simulink model "controlMCUSlugsMKII"  (Simulink 6.6)
settings: Solver=FixedStepDiscrete  StartTime=0.0  StopTime=10.0  FixedStep=0.01  RelTol=1e-3
InitFcn:
  | mcuInit
values from neighbouring files (symbols this model uses):
  apSampleTime = 0.01    [mcuInit.m]
  derivativesConstant = 5    [mcuInit.m]
  T = 0.01    [mcuInit.m]
undefined symbols (not defined in the file or in its folder): bankCommandLimit, baseHeight, bda, bde, bdr, bdt, bICda, bICde, bICdr, bICdt, controlMCUInit, daLimit, deLimit, drLimit, dtLimit, getAccBias, getAccels, getAttitude, getMidLevelCommands, getPassValues, getPidIdx, getVned, getWP, getXYZ, gsRead, ISA_g, lowRateTelemetryMavlink, mda, mde, mdr, mdt, mICda, mICde, mICdr, mICdt, pitchCommandLimit, protDecodeMavlink, readIpc, send2GS, setCurrentCommands, setDiagnosticFloat, setDiagnosticShort, setLogFloat1, setLogFloat2, setNavLat, setNavLong, setNavNav, u1, u2, updateEuler, updateLoad, updatePQR, updatePWM, updatePWM2, y1
libraries: dsPICdrivers x85, simulink x79, SLUGS_Library x23, aerolibconvert2 x5, aerolibutil x3
(part 1 of 5)
settings Model: Creator=ASL_Lab  LastModifiedBy=Administrator  ProdHWDeviceType=16-bit Generic
settings OptimizationCC: InlineParams=on  OptimizeModelRefInitCode=on  LifeSpan=1
settings HardwareCC: ProdBitPerInt=16  ProdEndianess=LittleEndian  ProdWordSize=16  ProdHWDeviceType=16-bit Generic  TargetHWDeviceType=32-bit Generic
settings RTWCC: SystemTargetFile=dspic.tlc  TemplateMakefile=dspic_pic30_gcc.tmf  PostCodeGenCommand=dsPIC_Compile()  Description=Embedded Target for Microchip dsPIC (real-time)  GenerateReport=on  ProcessScript=dspic_make_rtw_hook  CustomInclude=..\mavlink\include\slugs\  IncludeHyperlinkInReport=on  LaunchReport=on
settings RTWCC: CustomSource=|
  | clib\circBuffer.c
  | clib\sbrk.c
  | clib\interProcCommSlave.c
  | clib\eepLoader.c
  | clib\apUtils.c
  | clib\DEE.c
  | clib\DEES.s
  | clib\navSupport.c
  | clib\mavlinkControlMcu.c
  | clib\updateControlMcuState.c
  | clib\mavlinkCommsControlMcu.c
settings CodeAppCC: IgnoreCustomStorageClasses=off
settings STFCustomTargetCC: TargetFcnLib=ansi_tfl_tmw.mat  GenFloatMathFcnCalls=ANSI_C  ModelReferenceCompliant=off  IncludeMdlTerminateFcn=off  CombineOutputUpdateFcns=on  SuppressErrorStatus=on  ERTCustomFileBanners=on  SupportContinuousTime=off  SupportNonInlinedSFcns=off  SystemTargetFile=dspic.tlc
settings ERTTargetCC: TargetFcnLib=ansi_tfl_tmw.mat  GenFloatMathFcnCalls=ANSI_C  ModelReferenceCompliant=off  IncludeMdlTerminateFcn=off  SuppressErrorStatus=on  ModelStepFunctionPrototypeControlCompliant=off  ExtModeMexFile=noextcomm  InlinedParameterPlacement=NonHierarchical  ERTSrcFileBannerTemplate=dsPIC_code_template.cgt  ERTHdrFileBannerTemplate=dsPIC_code_template.cgt  ERTDataSrcFileTemplate=dsPIC_code_template.cgt  ERTDataHdrFileTemplate=dsPIC_code_template.cgt  ERTCustomFileTemplate=dsPIC_main.tlc
settings CustomProperty: DataType=string  Value=C:\PROGRA~1\MATLAB\R2007a\rtw\bin\win32\gmake

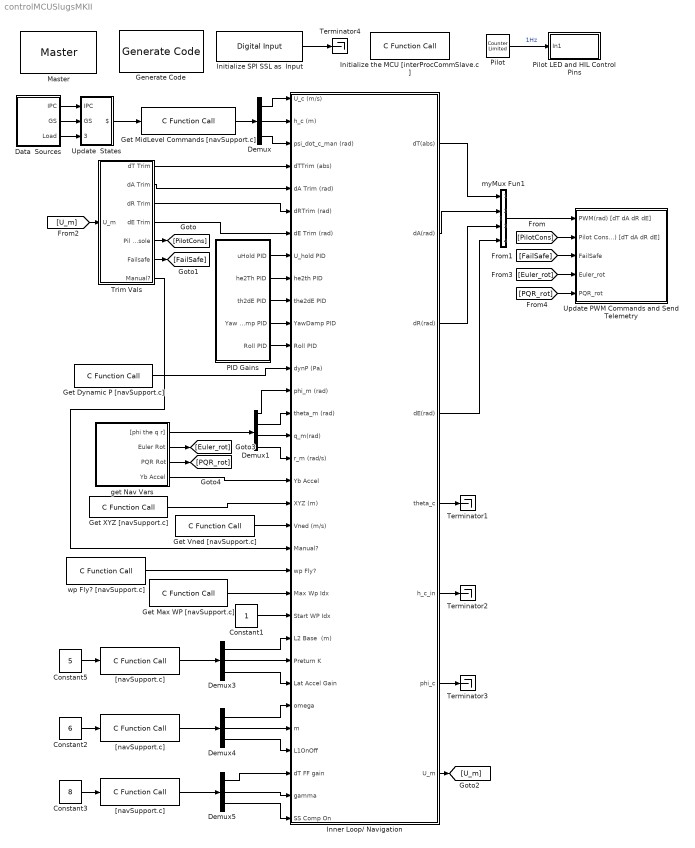
== system controlMCUSlugsMKII ==
  Constant1 : Constant  OutDataTypeMode=uint8
  Constant2 : Constant  Value=6  OutDataTypeMode=uint8
  Constant3 : Constant  Value=8  OutDataTypeMode=uint8
  Constant5 : Constant  Value=5  OutDataTypeMode=uint8
  Data  Sources : Subsystem
  Demux{,3..5} (4 alike) : Demux  Outputs=3
  Demux1 : Demux
  Generate Code : dsPICdrivers/Simulink Configuration/Generate Code
  Get Dynamic P [navSupport.c] : dsPICdrivers/OTHERS/C Function Call  Tag=dsPIC_dsPIC_CFunctionCall  fctName='getDynamic'  INPUT_SIZE=1  INPUT1=--  INPUT2=--  INPUT3=--  OUTPUT_SIZE=1  OUTPUT1=real32  SampleTime=.01  InputType=[ ]  OutputType=[ 7 ]  FctDeclaration=extern real32_T getDynamic();  FctCall=%y1 = getDynamic();  OrderingInOutPopup=None
  Get Max WP [navSupport.c] : dsPICdrivers/OTHERS/C Function Call  Tag=dsPIC_dsPIC_CFunctionCall  fctName='getMaxWp'  INPUT_SIZE=1  INPUT1=--  INPUT2=--  INPUT3=--  OUTPUT_SIZE=1  OUTPUT1=uint8  SampleTime=.01  InputType=[ ]  OutputType=[ 2 ]  FctDeclaration=extern uint8_T getMaxWp();  FctCall=%y1 = getMaxWp();  OrderingInOutPopup=None
  Get MidLevel Commands [navSupport.c] : dsPICdrivers/OTHERS/C Function Call  Tag=dsPIC_dsPIC_CFunctionCall  fctName='getMidLevelCommands'  INPUT_SIZE=1  INPUT1=--  INPUT2=--  INPUT3=--  OUTPUT_SIZE=3  OUTPUT1=real32  SampleTime=.01  InputType=[ ]  OutputType=[ 7 ]  FctDeclaration=extern void getMidLevelCommands(real32_T* y1);  FctCall=getMidLevelCommands(*%y1);  OrderingInOutPopup=Input
  Get Vned [navSupport.c] : dsPICdrivers/OTHERS/C Function Call  Tag=dsPIC_dsPIC_CFunctionCall  fctName='getVned'  INPUT_SIZE=1  INPUT1=--  INPUT2=--  INPUT3=--  OUTPUT_SIZE=3  OUTPUT1=real32  SampleTime=.01  InputType=[ ]  OutputType=[ 7 ]  FctDeclaration=extern void getVned(real32_T* y1);  FctCall=getVned(*%y1);  OrderingInOutPopup=None
  Get XYZ [navSupport.c] : dsPICdrivers/OTHERS/C Function Call  Tag=dsPIC_dsPIC_CFunctionCall  fctName='getXYZ'  INPUT_SIZE=1  INPUT1=--  INPUT2=--  INPUT3=--  OUTPUT_SIZE=3  OUTPUT1=real32  SampleTime=.01  InputType=[ ]  OutputType=[ 7 ]  FctDeclaration=extern void getXYZ(real32_T* y1);  FctCall=getXYZ(*%y1);  OrderingInOutPopup=None
  Initialize SPI SSL as  Input : dsPICdrivers/Digital I//O/Digital Input  Tag=dsPIC_Digital_Input  PORT=B  Pin=[2]  SampleTime=inf  OrderingInOutPopup=None
  Initialize the MCU [interProcCommSlave.c] : dsPICdrivers/OTHERS/C Function Call  Tag=dsPIC_dsPIC_CFunctionCall  fctName='controlMCUInit'  INPUT_SIZE=1  INPUT1=--  INPUT2=--  INPUT3=--  OUTPUT_SIZE=1  OUTPUT1=--  SampleTime=inf  InputType=[ ]  OutputType=[ ]  FctDeclaration=extern void controlMCUInit();  FctCall=controlMCUInit();  OrderingInOutPopup=None
  Inner Loop/ Navigation : Subsystem
  Master : dsPICdrivers/Master  Tag=dsPIC_MASTER  Priority=1  TimeStepType=Timer1  picType=33fJ256MC710  fcy=40000000  Quartz_33f=12e6  PLLActive_33f=on  fcyDesired_33f=40e6  tmr1="[8  49999  0]"  tmr1Info="Time Step : 0.01  ;   Error : 0%  PR1=49999"  tmr2345="[8  0  0  0  0  0  0  0]"  tmr2345cfg=[-1 -1 -1 -1 -1 -1 -1 -1]  IOautoConf=on  typePort="[ 0   0   0   0   0   0   0   0   0   0   0   0   0   0   0   0   0   0   9   0   0   0  10   0   0   0   0   0   0   0   0   0   0   0   0   0   0   0   0   0   0   0   0   0   0   0   0   0   0   0   0   0   0   0   0   0   0   6   6   6   6   0   0   6  11   0  11   0  11   0  11   0   0  10   0   0   0   0   0   0   0   0   0   0   0   0   0   0   0   0   0   0   0   0   0   0   0   0   0   0   0   0   0   0   0   0   0   0   0   0   0   0 ]"  TRIS="[ 65535  65471  65535  65535  65023  65535  65535 ]"  ADPCFG=2097220  MasterBusyPort=None  MasterOverloadPort=None  FOSC=External Clock  ClockSwitchMonitor=Both disabled  TempProtection_33f=TEMP_ON  FPBOR=<empty>  PWRT=64ms  MCLR=<empty>  PowerSave=off  OverrideFcy=off  NewFcy=1e6  PR2345="[65535  65535  65535  65535  65535  65535  65535  65535]"
  PID Gains : Subsystem
  Pilot : simulink/Sources/Counter Limited  SystemSampleTime=-1  uplimit=1  tsamp=1.0
  Pilot LED and HIL Control Pins : Subsystem
  Terminator{1..4} (4 alike) : Terminator
  Trim Vals : Subsystem
  Update  States : Subsystem
  Update PWM Commands and Send Telemetry : Subsystem
  "[navSupport.c]" : dsPICdrivers/OTHERS/C Function Call  Tag=dsPIC_dsPIC_CFunctionCall  fctName='getPidIdx'  INPUT_SIZE=1  INPUT1=uint8  INPUT2=--  INPUT3=--  OUTPUT_SIZE=3  OUTPUT1=real32  SampleTime=.01  InputType=[ 2 ]  OutputType=[ 7 ]  FctDeclaration=extern void getPidIdx(uint8_T u1,real32_T* y1);  FctCall=getPidIdx(%u1, *%y1);  OrderingInOutPopup=None
  "[navSupport.c] " : dsPICdrivers/OTHERS/C Function Call  Tag=dsPIC_dsPIC_CFunctionCall  fctName='getPidIdx'  INPUT_SIZE=1  INPUT1=uint8  INPUT2=--  INPUT3=--  OUTPUT_SIZE=3  OUTPUT1=real32  SampleTime=.01  InputType=[ 2 ]  OutputType=[ 7 ]  FctDeclaration=extern void getPidIdx(uint8_T u1,real32_T* y1);  FctCall=getPidIdx(%u1, *%y1);  OrderingInOutPopup=None
  "[navSupport.c]   " : dsPICdrivers/OTHERS/C Function Call  Tag=dsPIC_dsPIC_CFunctionCall  fctName='getPidIdx'  INPUT_SIZE=1  INPUT1=uint8  INPUT2=--  INPUT3=--  OUTPUT_SIZE=3  OUTPUT1=real32  SampleTime=.01  InputType=[ 2 ]  OutputType=[ 7 ]  FctDeclaration=extern void getPidIdx(uint8_T u1,real32_T* y1);  FctCall=getPidIdx(%u1, *%y1);  OrderingInOutPopup=None
  get Nav Vars : Subsystem
  myMux Fun1 : Stateflow chart
  wp Fly? [navSupport.c] : dsPICdrivers/OTHERS/C Function Call  Tag=dsPIC_dsPIC_CFunctionCall  fctName='isWpFly'  INPUT_SIZE=1  INPUT1=--  INPUT2=--  INPUT3=--  OUTPUT_SIZE=1  OUTPUT1=uint8  SampleTime=.01  InputType=[ ]  OutputType=[ 2 ]  FctDeclaration=extern uint8_T isWpFly();  FctCall=%y1 = isWpFly();  OrderingInOutPopup=None
  wires:
  Pilot/1 -> Pilot LED and HIL Control Pins/1(In1)  "1Hz"
  Initialize SPI SSL as  Input/1 -> Terminator4/1
  Data  Sources/1(IPC) -> Update  States/1(IPC)
  Data  Sources/2(GS) -> Update  States/2(GS)
  Data  Sources/3(Load) -> Update  States/3(Load)
  Demux/1 -> Inner Loop/ Navigation/1(U_c (m/s))
  Demux/2 -> Inner Loop/ Navigation/2(h_c (m))
  Demux/3 -> Inner Loop/ Navigation/3(psi_dot_c_man (rad))
  Get MidLevel Commands [navSupport.c]/1 -> Demux/1
  Trim Vals/4(dE Trim) -> Inner Loop/ Navigation/7(dE Trim (rad))
  Trim Vals/1(dT Trim) -> Inner Loop/ Navigation/4(dTTrim (abs))
  Trim Vals/2(dA Trim) -> Inner Loop/ Navigation/5(dA Trim (rad))
  Trim Vals/3(dR Trim) -> Inner Loop/ Navigation/6(dRTrim (rad))
  PID Gains/1(uHold PID) -> Inner Loop/ Navigation/8(U_hold PID)
  PID Gains/2(he2Th PID) -> Inner Loop/ Navigation/9(he2th PID)
  PID Gains/3(th2dE PID) -> Inner Loop/ Navigation/10(the2dE PID)
  PID Gains/4(Yaw Damp PID) -> Inner Loop/ Navigation/11(YawDamp PID)
  PID Gains/5(Roll PID) -> Inner Loop/ Navigation/12("Roll PID ")
  Constant1/1 -> Inner Loop/ Navigation/24(Start WP Idx)
  Get Dynamic P [navSupport.c]/1 -> Inner Loop/ Navigation/13(dynP (Pa))
  get Nav Vars/1("[phi the q r]") -> Demux1/1
  Demux1/1 -> Inner Loop/ Navigation/14(phi_m (rad))
  Demux1/2 -> Inner Loop/ Navigation/15(theta_m (rad))
  Get Max WP [navSupport.c]/1 -> Inner Loop/ Navigation/23(Max Wp Idx)
  Update  States/1($) -> Get MidLevel Commands [navSupport.c]/1
  Trim Vals/7(Manual?) -> Inner Loop/ Navigation/21(Manual?)
  wp Fly? [navSupport.c]/1 -> Inner Loop/ Navigation/22(wp Fly?)
  Inner Loop/ Navigation/5(theta_c) -> Terminator1/1
  Inner Loop/ Navigation/6(h_c_in) -> Terminator2/1
  Inner Loop/ Navigation/7(phi_c) -> Terminator3/1
  Constant5/1 -> "[navSupport.c]"/1
  "[navSupport.c]"/1 -> Demux3/1
  Demux3/1 -> Inner Loop/ Navigation/25(L2 Base  (m))
  Demux3/2 -> Inner Loop/ Navigation/26(Preturn K)
  Demux1/4 -> Inner Loop/ Navigation/17(r_m (rad/s))
  Demux1/3 -> Inner Loop/ Navigation/16(q_m(rad))
  Demux3/3 -> Inner Loop/ Navigation/27(Lat Accel Gain)
  Constant2/1 -> "[navSupport.c] "/1
  "[navSupport.c] "/1 -> Demux4/1
  Demux4/1 -> Inner Loop/ Navigation/28(omega)
  Demux4/2 -> Inner Loop/ Navigation/29(m)
  Demux4/3 -> Inner Loop/ Navigation/30(L1OnOff)
  Trim Vals/5(Pil Console) -> [PilotCons]
  Trim Vals/6("Failsafe ") -> [FailSafe]
  Inner Loop/ Navigation/1(dT(abs)) -> myMux Fun1/1(u1)
  Inner Loop/ Navigation/2(dA(rad)) -> myMux Fun1/2(u2)
  Inner Loop/ Navigation/3(dR(rad)) -> myMux Fun1/3(u3)
  Inner Loop/ Navigation/4(dE(rad)) -> myMux Fun1/4(u4)
  [PilotCons] -> Update PWM Commands and Send Telemetry/2(Pilot Console (IC) [dT dA dR dE])
  myMux Fun1/1(y) -> Update PWM Commands and Send Telemetry/1(PWM(rad) [dT dA dR dE])
  Inner Loop/ Navigation/8(U_m) -> [U_m]
  [U_m] -> Trim Vals/1(U_m)
  [FailSafe] -> Update PWM Commands and Send Telemetry/3(FailSafe)
  get Nav Vars/2(Euler Rot) -> [Euler_rot]
  get Nav Vars/3(PQR Rot) -> [PQR_rot]
  [Euler_rot] -> Update PWM Commands and Send Telemetry/4(Euler_rot)
  [PQR_rot] -> Update PWM Commands and Send Telemetry/5(PQR_rot)
  Constant3/1 -> "[navSupport.c]   "/1
  "[navSupport.c]   "/1 -> Demux5/1
  Demux5/1 -> Inner Loop/ Navigation/31(dT FF gain)
  Demux5/2 -> Inner Loop/ Navigation/32(gamma)
  Demux5/3 -> Inner Loop/ Navigation/33(SS Comp On)
  get Nav Vars/4(Yb Accel) -> Inner Loop/ Navigation/18(Yb Accel)
  Get XYZ [navSupport.c]/1 -> Inner Loop/ Navigation/19(XYZ (m))
  Get Vned [navSupport.c]/1 -> Inner Loop/ Navigation/20(Vned (m/s))

== system controlMCUSlugsMKII/Data  Sources ==
  Compute Load : Subsystem
  Data from GS [mavlinkCommsControlMcu.c] : dsPICdrivers/OTHERS/C Function Call  Tag=dsPIC_dsPIC_CFunctionCall  fctName='gsRead'  INPUT_SIZE=1  INPUT1=--  INPUT2=--  INPUT3=--  OUTPUT_SIZE=109  OUTPUT1=uint8  SampleTime=.01  InputType=[ ]  OutputType=[ 2 ]  FctDeclaration=extern void gsRead(uint8_T* y1);  FctCall=gsRead(*%y1);  OrderingInOutPopup=None
  Data from IPC [interProcCommSlave.c] : dsPICdrivers/OTHERS/C Function Call  Tag=dsPIC_dsPIC_CFunctionCall  fctName='readIpc'  INPUT_SIZE=1  INPUT1=--  INPUT2=--  INPUT3=--  OUTPUT_SIZE=109  OUTPUT1=uint8  SampleTime=.01  InputType=[ ]  OutputType=[ 2 ]  FctDeclaration=extern void readIpc(uint8_T* y1);  FctCall=readIpc(*%y1);  OrderingInOutPopup=None
  IPC : Outport
  GS : Outport  Port=2
  Load : Outport  Port=3
  wires:
  Data from IPC [interProcCommSlave.c]/1 -> IPC/1
  Data from GS [mavlinkCommsControlMcu.c]/1 -> GS/1
  Compute Load/1(Load (%)) -> Load/1

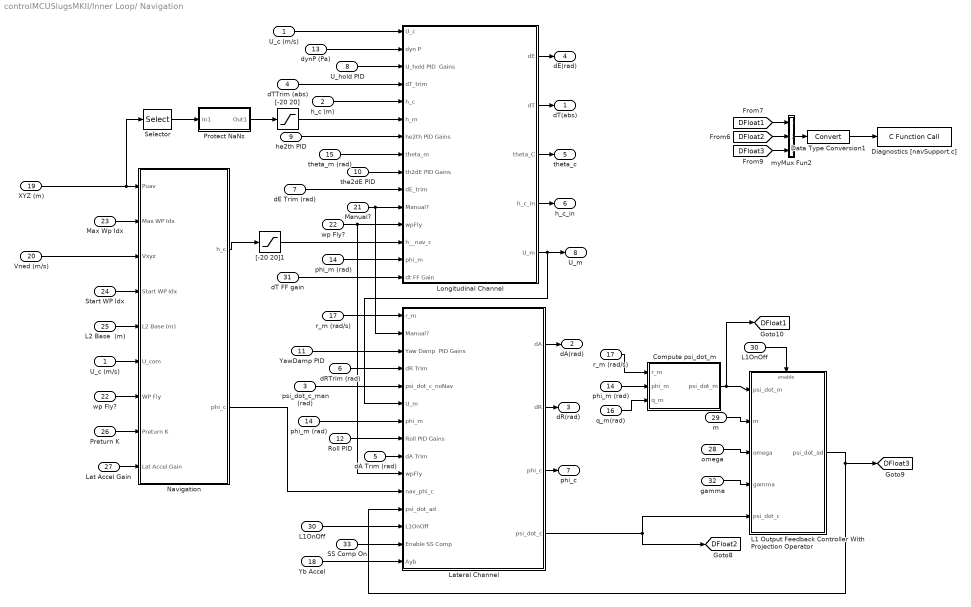
== system controlMCUSlugsMKII/Inner Loop/ Navigation ==
  U_c (m/s) : Inport
  h_c (m) : Inport  Port=2
  psi_dot_c_man (rad) : Inport  Port=3
  dTTrim (abs) : Inport  Port=4
  dA Trim (rad) : Inport  Port=5
  dRTrim (rad) : Inport  Port=6
  dE Trim (rad) : Inport  Port=7
  U_hold PID : Inport  Port=8
  he2th PID : Inport  Port=9
  the2dE PID : Inport  Port=10
  YawDamp PID : Inport  Port=11
  "Roll PID " : Inport  Port=12
  dynP (Pa) : Inport  Port=13
  phi_m (rad) : Inport  Port=14
  theta_m (rad) : Inport  Port=15
  q_m(rad) : Inport  Port=16
  r_m (rad/s) : Inport  Port=17
  Yb Accel : Inport  Port=18
  XYZ (m) : Inport  Port=19
  Vned (m/s) : Inport  Port=20
  Manual? : Inport  Port=21
  wp Fly? : Inport  Port=22
  Max Wp Idx : Inport  Port=23
  Start WP Idx : Inport  Port=24
  L2 Base  (m) : Inport  Port=25
  Preturn K : Inport  Port=26
  Lat Accel Gain : Inport  Port=27
  omega : Inport  Port=28
  m : Inport  Port=29
  L1OnOff : Inport  Port=30
  dT FF gain : Inport  Port=31
  gamma : Inport  Port=32
  SS Comp On : Inport  Port=33
  Compute psi_dot_m : Subsystem
  Data Type Conversion1 : DataTypeConversion  OutDataTypeMode=single
  Diagnostics [navSupport.c] : dsPICdrivers/OTHERS/C Function Call  Tag=dsPIC_dsPIC_CFunctionCall  fctName='setDiagnosticFloat'  INPUT_SIZE=3  INPUT1=real32  INPUT2=--  INPUT3=--  OUTPUT_SIZE=1  OUTPUT1=--  SampleTime=.01  InputType=[ 7 ]  OutputType=[ ]  FctDeclaration=extern void setDiagnosticFloat(real32_T* u1);  FctCall=setDiagnosticFloat(*%u1);  OrderingInOutPopup=None
  L1 Output Feedback Controller With  Projection Operator : Subsystem  TreatAsAtomicUnit=on
  "L1OnOff " : InportShadow  Port=30  LatchByCopyingInsideSignal=off
  Lateral Channel : Subsystem  AncestorBlock=SLUGS_Library/InnerLoop/Lateral Channel  TreatAsAtomicUnit=on
  Longitudinal Channel : Subsystem  AncestorBlock=SLUGS_Library/InnerLoop/Longitudinal Channel  TreatAsAtomicUnit=on
  Navigation : Subsystem  Priority=13  AncestorBlock=SLUGS_Library/InnerLoop/Navigation  TreatAsAtomicUnit=on
  Protect NaNs : Subsystem
  Selector : Selector  IndexOptions=Index vector (dialog)  Indices=[3]  OutputSizes=1  InputPortWidth=3
  "U_c (m/s) " : InportShadow  Port=1  LatchByCopyingInsideSignal=off
  "[-20 20]" : Saturate  UpperLimit=350  LowerLimit=170
  "[-20 20]1" : Saturate  UpperLimit=350  LowerLimit=170
  myMux Fun2 : Stateflow chart
  "phi_m (rad) " : InportShadow  Port=14  LatchByCopyingInsideSignal=off
  "phi_m (rad)   " : InportShadow  Port=14  LatchByCopyingInsideSignal=off
  "r_m (rad/s) " : InportShadow  Port=17  LatchByCopyingInsideSignal=off
  "wp Fly? " : InportShadow  Port=22  LatchByCopyingInsideSignal=off
  dT(abs) : Outport
  dA(rad) : Outport  Port=2
  dR(rad) : Outport  Port=3
  dE(rad) : Outport  Port=4
  theta_c : Outport  Port=5
  h_c_in : Outport  Port=6
  phi_c : Outport  Port=7
  U_m : Outport  Port=8
  tag scope: DFloat1=global, DFloat2=global, DFloat3=global
  wires:
  Manual?/1 -> Longitudinal Channel/11(Manual?), Lateral Channel/2(Manual?)
  wp Fly?/1 -> Longitudinal Channel/12(wpFly), Lateral Channel/10(wpFly)
  U_c (m/s)/1 -> Longitudinal Channel/1(U_c)
  dynP (Pa)/1 -> Longitudinal Channel/2(dyn P)
  Longitudinal Channel/1(dE) -> dE(rad)/1
  U_hold PID/1 -> Longitudinal Channel/3(U_hold PID  Gains)
  dTTrim (abs)/1 -> Longitudinal Channel/4(dT_trim)
  h_c (m)/1 -> Longitudinal Channel/5(h_c)
  Longitudinal Channel/2(dT) -> dT(abs)/1
  Selector/1 -> Protect NaNs/1(In1)
  he2th PID/1 -> Longitudinal Channel/7(he2th PID Gains)
  theta_m (rad)/1 -> Longitudinal Channel/8(theta_m)
  Longitudinal Channel/3(theta_C) -> theta_c/1
  the2dE PID/1 -> Longitudinal Channel/9(th2dE PID Gains)
  dE Trim (rad)/1 -> Longitudinal Channel/10(dE_trim)
  Longitudinal Channel/4(h_c_in) -> h_c_in/1
  r_m (rad/s)/1 -> Lateral Channel/1(r_m)
  YawDamp PID/1 -> Lateral Channel/3(Yaw Damp  PID Gains)
  dRTrim (rad)/1 -> Lateral Channel/4(dR Trim)
  Lateral Channel/2(dR) -> dR(rad)/1
  psi_dot_c_man (rad)/1 -> Lateral Channel/5(psi_dot_c_noNav)
  phi_m (rad)/1 -> Lateral Channel/7(phi_m)
  Lateral Channel/3(phi_c) -> phi_c/1
  "Roll PID "/1 -> Lateral Channel/8(Roll PID Gains)
  dA Trim (rad)/1 -> Lateral Channel/9(dA Trim)
  Longitudinal Channel/5(U_m) -> Lateral Channel/6(U_m), U_m/1
  XYZ (m)/1 -> Selector/1, Navigation/1(Puav)
  Max Wp Idx/1 -> Navigation/2(Max WP Idx)
  Vned (m/s)/1 -> Navigation/3(Vxyz)
  Start WP Idx/1 -> Navigation/4(Start WP Idx)
  L2 Base  (m)/1 -> Navigation/5(L2 Base (m))
  Navigation/1(h_c) -> "[-20 20]1"/1
  Navigation/2(phi_c) -> Lateral Channel/11(nav_phi_c)
  Compute psi_dot_m/1(psi_dot_m) -> L1 Output Feedback Controller With  Projection Operator/1(psi_dot_m), [DFloat1]
  m/1 -> L1 Output Feedback Controller With  Projection Operator/2(m)
  omega/1 -> L1 Output Feedback Controller With  Projection Operator/3(omega)
  gamma/1 -> L1 Output Feedback Controller With  Projection Operator/4(gamma)
  "r_m (rad/s) "/1 -> Compute psi_dot_m/1(r_m)
  "phi_m (rad) "/1 -> Compute psi_dot_m/2(phi_m)
  q_m(rad)/1 -> Compute psi_dot_m/3(q_m)
  L1OnOff/1 -> L1 Output Feedback Controller With  Projection Operator/Enable
  L1 Output Feedback Controller With  Projection Operator/1(psi_dot_ad) -> Lateral Channel/12(psi_dot_ad), [DFloat3]
  "L1OnOff "/1 -> Lateral Channel/13(L1OnOff)
  "U_c (m/s) "/1 -> Navigation/6(U_com)
  Preturn K/1 -> Navigation/8(Preturn K)
  "phi_m (rad)   "/1 -> Longitudinal Channel/14(phi_m)
  "wp Fly? "/1 -> Navigation/7(WP Fly)
  dT FF gain/1 -> Longitudinal Channel/15(dt FF Gain)
  Lateral Channel/1(dA) -> dA(rad)/1
  Lat Accel Gain/1 -> Navigation/9(Lat Accel Gain)
  SS Comp On/1 -> Lateral Channel/14(Enable SS Comp)
  Yb Accel/1 -> Lateral Channel/15(Ayb)
  Lateral Channel/4("psi_dot_c ") -> L1 Output Feedback Controller With  Projection Operator/5(psi_dot_c), [DFloat2]
  Protect NaNs/1(Out1) -> "[-20 20]"/1
  "[-20 20]"/1 -> Longitudinal Channel/6(h_m)
  "[-20 20]1"/1 -> Longitudinal Channel/13(h__nav_c)
  [DFloat1] -> myMux Fun2/1(u1)
  [DFloat2] -> myMux Fun2/2(u2)
  [DFloat3] -> myMux Fun2/3(u3)
  myMux Fun2/1(y) -> Data Type Conversion1/1
  Data Type Conversion1/1 -> Diagnostics [navSupport.c]/1

== system controlMCUSlugsMKII/PID Gains ==
  Constant1 : Constant  Value=0  OutDataTypeMode=uint8
  Constant2 : Constant  OutDataTypeMode=uint8
  Constant3 : Constant  Value=2  OutDataTypeMode=uint8
  Constant4 : Constant  Value=3  OutDataTypeMode=uint8
  Constant5 : Constant  Value=4  OutDataTypeMode=uint8
  Get Pid according to Index{,1..3} (4 alike) : dsPICdrivers/OTHERS/C Function Call  Tag=dsPIC_dsPIC_CFunctionCall  fctName='getPidIdx'  INPUT_SIZE=1  INPUT1=uint8  INPUT2=--  INPUT3=--  OUTPUT_SIZE=3  OUTPUT1=real32  SampleTime=.01  InputType=[ 2 ]  OutputType=[ 7 ]  FctDeclaration=extern void getPidIdx(uint8_T u1,real32_T* y1);  FctCall=getPidIdx(%u1, *%y1);  OrderingInOutPopup=None
  "[navSupport.c]" : dsPICdrivers/OTHERS/C Function Call  Tag=dsPIC_dsPIC_CFunctionCall  fctName='getPidIdx'  INPUT_SIZE=1  INPUT1=uint8  INPUT2=--  INPUT3=--  OUTPUT_SIZE=3  OUTPUT1=real32  SampleTime=.01  InputType=[ 2 ]  OutputType=[ 7 ]  FctDeclaration=extern void getPidIdx(uint8_T u1,real32_T* y1);  FctCall=getPidIdx(%u1, *%y1);  OrderingInOutPopup=None
  uHold PID : Outport
  he2Th PID : Outport  Port=2
  th2dE PID : Outport  Port=3
  Yaw Damp PID : Outport  Port=4
  Roll PID : Outport  Port=5
  wires:
  Constant1/1 -> Get Pid according to Index/1
  Constant2/1 -> Get Pid according to Index1/1
  Constant3/1 -> Get Pid according to Index2/1
  Constant4/1 -> Get Pid according to Index3/1
  Constant5/1 -> "[navSupport.c]"/1
  Get Pid according to Index/1 -> uHold PID/1
  Get Pid according to Index1/1 -> he2Th PID/1
  Get Pid according to Index2/1 -> th2dE PID/1
  Get Pid according to Index3/1 -> Yaw Damp PID/1
  "[navSupport.c]"/1 -> Roll PID/1

== system controlMCUSlugsMKII/Pilot LED and HIL Control Pins ==
  In1 : Inport
  Data Type Conversion1 : DataTypeConversion  OutDataTypeMode=boolean
  Data Type Conversion2 : DataTypeConversion  OutDataTypeMode=boolean
  HIL Attitude  On/Off Switch : dsPICdrivers/Digital I//O/Digital Output Write  Tag=dsPIC_Digital_Output  Priority=5  PORT=B  Pin=[6]  Simultaneous=off  OrderingInOutPopup=None
  HIL On/Off Switch : dsPICdrivers/Digital I//O/Digital Output Write  Tag=dsPIC_Digital_Output  Priority=5  PORT=E  Pin=[9]  Simultaneous=off  OrderingInOutPopup=None
  Put getHilOnOff function here : Constant  Value=0  OutDataTypeMode=uint8
  Terminator : Terminator
  wires:
  Put getHilOnOff function here/1 -> Data Type Conversion1/1
  Data Type Conversion1/1 -> HIL On/Off Switch/1, HIL Attitude  On/Off Switch/1
  In1/1 -> Data Type Conversion2/1
  Data Type Conversion2/1 -> Terminator/1

== system controlMCUSlugsMKII/Trim Vals ==
  U_m : Inport  Orientation=left
  Abs{,1..2,4} (4 alike) : Abs
  Bufffer IC : Subsystem
  Control Surfaces [dT dA dR dE] : Selector  IndexOptions=Index vector (dialog)  Indices=[1 2 4 3]  OutputSizes=1  InputPortWidth=5
  Control Surface Input : Subsystem
  Detect Transition High to Low : Subsystem
  Failsafe : Selector  Orientation=left  IndexOptions=Index vector (dialog)  Indices=5  OutputSizes=1  InputPortWidth=5
  Gain1 : Gain  Gain=(180/pi)*100
  Gain2 : Gain  Gain=(180/pi)*100
  Gain3 : Gain  Gain=(180/pi)*100
  Gain4 : Gain  Gain=100
  Grab I.C. : Subsystem  TreatAsAtomicUnit=on
  Integer Delay : simulink/Discrete/Integer Delay  Orientation=left  vinit=0.0  samptime=.01  NumDelays=1
  Log  Trims Using PWM High [groundStationDriver.c] : Subsystem
  Manual or Auto? [navSupport.c] : dsPICdrivers/OTHERS/C Function Call  Tag=dsPIC_dsPIC_CFunctionCall  fctName='isApManual'  INPUT_SIZE=1  INPUT1=--  INPUT2=--  INPUT3=--  OUTPUT_SIZE=1  OUTPUT1=uint8  SampleTime=.01  InputType=[ ]  OutputType=[ 2 ]  FctDeclaration=extern uint8_T isApManual();  FctCall=%y1 = isApManual();  OrderingInOutPopup=None
  dT Trim : Outport
  dA Trim : Outport  Port=2
  dR Trim : Outport  Port=3
  dE Trim : Outport  Port=4
  Pil Console : Outport  Port=5
  "Failsafe " : Outport  Orientation=left  Port=6
  Manual? : Outport  Orientation=left  Port=7
  wires:
  Manual or Auto? [navSupport.c]/1 -> Detect Transition High to Low/1(Switch), Manual?/1
  Control Surface Input/1(Pilot Console) -> Control Surfaces [dT dA dR dE]/1, Failsafe/1
  Control Surfaces [dT dA dR dE]/1 -> Pil Console/1, Bufffer IC/1(Pilot Console)
  Failsafe/1 -> "Failsafe "/1
  Gain1/1 -> Abs/1
  Gain2/1 -> Abs2/1
  Gain3/1 -> Abs1/1
  Abs/1 -> Log  Trims Using PWM High [groundStationDriver.c]/2(In2)
  Abs1/1 -> Log  Trims Using PWM High [groundStationDriver.c]/3(In3)
  Abs2/1 -> Log  Trims Using PWM High [groundStationDriver.c]/4(In4)
  U_m/1 -> Integer Delay/1
  Integer Delay/1 -> Grab I.C./5(U_m)
  Bufffer IC/1(dT_buf) -> Grab I.C./1(dT_buf)
  Bufffer IC/2(dA_buf) -> Grab I.C./2(dA_buf)
  Bufffer IC/3(dR_buf) -> Grab I.C./3(dR_buf)
  Bufffer IC/4(dE_buf) -> Grab I.C./4(dE_buf)
  Grab I.C./4(dE_trim) -> dE Trim/1, Gain3/1
  Grab I.C./3(dR_trim) -> dR Trim/1, Gain2/1
  Grab I.C./2(dA_trim) -> dA Trim/1, Gain1/1
  Grab I.C./1(dT_trim) -> dT Trim/1, Gain4/1
  Detect Transition High to Low/1(Transition) -> Grab I.C./Enable
  Abs4/1 -> Log  Trims Using PWM High [groundStationDriver.c]/1(In1)
  Gain4/1 -> Abs4/1

== system controlMCUSlugsMKII/Update  States ==
  IPC : Inport
  GS : Inport  Port=2
  Load : Inport  Port=3
  GS Messages  Parser/Decoder [mavlinkCommsControlMcu.c] : dsPICdrivers/OTHERS/C Function Call  Tag=dsPIC_dsPIC_CFunctionCall  fctName='protDecodeMavlink'  INPUT_SIZE=109  INPUT1=uint8  INPUT2=--  INPUT3=--  OUTPUT_SIZE=1  OUTPUT1=--  SampleTime=-1  InputType=[ 2 ]  OutputType=[ ]  FctDeclaration=extern void protDecodeMavlink(uint8_T* u1);  FctCall=protDecodeMavlink(*%u1);  OrderingInOutPopup=Input & Output
  Parser/Decoder [mavlinkCommsControlMcu.c] : dsPICdrivers/OTHERS/C Function Call  Tag=dsPIC_dsPIC_CFunctionCall  fctName='protDecodeMavlink'  INPUT_SIZE=109  INPUT1=uint8  INPUT2=--  INPUT3=--  OUTPUT_SIZE=1  OUTPUT1=--  SampleTime=-1  InputType=[ 2 ]  OutputType=[ ]  FctDeclaration=extern void protDecodeMavlink(uint8_T* u1);  FctCall=protDecodeMavlink(*%u1);  OrderingInOutPopup=Output
  update Load of  Control MCU [updateControlMcu.c] : dsPICdrivers/OTHERS/C Function Call  Tag=dsPIC_dsPIC_CFunctionCall  fctName='updateLoad'  INPUT_SIZE=1  INPUT1=uint8  INPUT2=--  INPUT3=--  OUTPUT_SIZE=1  OUTPUT1=--  SampleTime=-1  InputType=[ 2 ]  OutputType=[ ]  FctDeclaration=extern void updateLoad(uint8_T u1);  FctCall=updateLoad(%u1);  OrderingInOutPopup=Input & Output
  $ : Outport
  wires:
  IPC/1 -> Parser/Decoder [mavlinkCommsControlMcu.c]/1
  GS/1 -> GS Messages  Parser/Decoder [mavlinkCommsControlMcu.c]/1
  Load/1 -> update Load of  Control MCU [updateControlMcu.c]/1
  Parser/Decoder [mavlinkCommsControlMcu.c]/1 -> GS Messages  Parser/Decoder [mavlinkCommsControlMcu.c]/2
  GS Messages  Parser/Decoder [mavlinkCommsControlMcu.c]/1 -> update Load of  Control MCU [updateControlMcu.c]/2
  update Load of  Control MCU [updateControlMcu.c]/1 -> $/1

== system controlMCUSlugsMKII/Update PWM Commands and Send Telemetry ==
  PWM(rad) [dT dA dR dE] : Inport
  Pilot Console (IC) [dT dA dR dE] : Inport  Port=2
  FailSafe : Inport  Port=3
  Euler_rot : Inport  Orientation=left  Port=4
  PQR_rot : Inport  Orientation=left  Port=5
  Create Telemetry  Sentence [mavlinkCommsControlMcu.c] : dsPICdrivers/OTHERS/C Function Call  Tag=dsPIC_dsPIC_CFunctionCall  fctName='lowRateTelemetryMavlink'  INPUT_SIZE=1  INPUT1=--  INPUT2=--  INPUT3=--  OUTPUT_SIZE=120  OUTPUT1=uint8  SampleTime=.01  InputType=[ ]  OutputType=[ 2 ]  FctDeclaration=extern void lowRateTelemetryMavlink(uint8_T* y1);  FctCall=lowRateTelemetryMavlink(*%y1);  OrderingInOutPopup=Input
  Demux : Demux
  Generate PWM Signals Based on the Control Type : Subsystem
  Get Control Type [navSupport.c] : dsPICdrivers/OTHERS/C Function Call  Tag=dsPIC_dsPIC_CFunctionCall  fctName='getApControlType'  INPUT_SIZE=1  INPUT1=--  INPUT2=--  INPUT3=--  OUTPUT_SIZE=1  OUTPUT1=uint8  SampleTime=.01  InputType=[ ]  OutputType=[ 2 ]  FctDeclaration=extern uint8_T getApControlType();  FctCall=%y1 = getApControlType();  OrderingInOutPopup=None
  PWM Servo Output : dsPICdrivers/Peripheral I//O/PWM Motor Output  Tag=dsPIC_PWM_Motor  Priority=5  InputEnableChk=off  InputPeriodeChk=off  Channel=[1 2 3 4]  TPeriode=.02  PrescalerValue=16  PeriodeInteger=25000  MaxName='PWM'  Centered=on  HChannelON=off  Info="Nbr Bits : 15.6096  ||  PWM = 50000  ||  Prescaler = 16"  Delay=0  IntPriority=5  nbrPwmChannelPIC=4  Status=OK
  Send Data to Radio Modem [mavlinkCommsControlMcu.c] : dsPICdrivers/OTHERS/C Function Call  Tag=dsPIC_dsPIC_CFunctionCall  fctName='send2GS'  INPUT_SIZE=120  INPUT1=uint8  INPUT2=--  INPUT3=--  OUTPUT_SIZE=1  OUTPUT1=--  SampleTime=-1  InputType=[ 2 ]  OutputType=[ ]  FctDeclaration=extern void send2GS(uint8_T* u1);  FctCall=send2GS(*%u1);  OrderingInOutPopup=None
  "Update PQR updateControlMcu.c] " : dsPICdrivers/OTHERS/C Function Call  Tag=dsPIC_dsPIC_CFunctionCall  fctName='updatePQR'  INPUT_SIZE=3  INPUT1=real32  INPUT2=--  INPUT3=--  OUTPUT_SIZE=1  OUTPUT1=--  SampleTime=.01  InputType=[ 7 ]  OutputType=[ ]  FctDeclaration=extern void updatePQR(real32_T* u1);  FctCall=updatePQR(*%u1);  OrderingInOutPopup=Input & Output
  Update PWM  Commands [updateControlMcu.c] : dsPICdrivers/OTHERS/C Function Call  Tag=dsPIC_dsPIC_CFunctionCall  fctName='updatePWM'  INPUT_SIZE=5  INPUT1=uint16  INPUT2=--  INPUT3=--  OUTPUT_SIZE=1  OUTPUT1=--  SampleTime=-1  InputType=[ 4 ]  OutputType=[ ]  FctDeclaration=extern void updatePWM(uint16_T* u1);  FctCall=updatePWM(*%u1);  OrderingInOutPopup=Output
  "Update the Euler Angles [updateControlMcu.c] " : dsPICdrivers/OTHERS/C Function Call  Tag=dsPIC_dsPIC_CFunctionCall  fctName='updateEuler'  INPUT_SIZE=3  INPUT1=real32  INPUT2=--  INPUT3=--  OUTPUT_SIZE=1  OUTPUT1=--  SampleTime=.01  InputType=[ 7 ]  OutputType=[ ]  FctDeclaration=extern void updateEuler(real32_T* u1);  FctCall=updateEuler(*%u1);  OrderingInOutPopup=Input & Output
  "[dR dE dA dT]" : Selector  IndexOptions=Index vector (dialog)  Indices=[3 4 2 1]  OutputSizes=1  InputPortWidth=4
  "[dR dE dA dT]2" : Selector  IndexOptions=Index vector (dialog)  Indices=2  OutputSizes=1  InputPortWidth=4
  "[dR dE dA dT]3" : Selector  IndexOptions=Index vector (dialog)  Indices=2  OutputSizes=1  InputPortWidth=4
  "[dT dA dE dR]" : Selector  Orientation=up  IndexOptions=Index vector (dialog)  Indices=[1 2 4 3 ]  OutputSizes=1  InputPortWidth=4
  myMux Fun1 : Stateflow chart
  wires:
  Create Telemetry  Sentence [mavlinkCommsControlMcu.c]/1 -> Send Data to Radio Modem [mavlinkCommsControlMcu.c]/1
  Get Control Type [navSupport.c]/1 -> Generate PWM Signals Based on the Control Type/1(Ctrl Type)
  "[dR dE dA dT]"/1 -> Demux/1
  Demux/1 -> PWM Servo Output/1
  Demux/2 -> PWM Servo Output/2
  Demux/3 -> PWM Servo Output/3
  Demux/4 -> PWM Servo Output/4
  Generate PWM Signals Based on the Control Type/1(PWM) -> "[dR dE dA dT]"/1, "[dT dA dE dR]"/1, "[dR dE dA dT]2"/1
  PWM(rad) [dT dA dR dE]/1 -> Generate PWM Signals Based on the Control Type/2(PWM(rad))
  Pilot Console (IC) [dT dA dR dE]/1 -> Generate PWM Signals Based on the Control Type/3(Pilot Console (IC))
  FailSafe/1 -> myMux Fun1/2(u2)
  myMux Fun1/1(y) -> Update PWM  Commands [updateControlMcu.c]/1
  "[dT dA dE dR]"/1 -> myMux Fun1/1(u1), "[dR dE dA dT]3"/1
  Euler_rot/1 -> "Update the Euler Angles [updateControlMcu.c] "/1
  PQR_rot/1 -> "Update PQR updateControlMcu.c] "/1
  Update PWM  Commands [updateControlMcu.c]/1 -> "Update the Euler Angles [updateControlMcu.c] "/2
  "Update the Euler Angles [updateControlMcu.c] "/1 -> "Update PQR updateControlMcu.c] "/2
  "Update PQR updateControlMcu.c] "/1 -> Create Telemetry  Sentence [mavlinkCommsControlMcu.c]/1

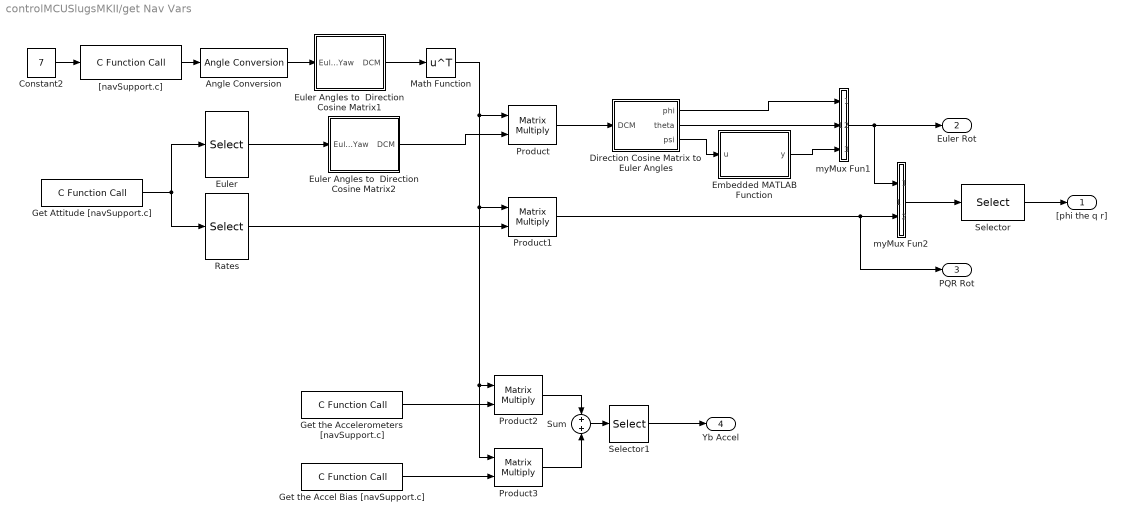
== system controlMCUSlugsMKII/get Nav Vars ==
  Angle Conversion : aerolibconvert2/Angle Conversion  SystemSampleTime=-1  IU=deg  OU=rad
  Constant2 : Constant  Value=7  OutDataTypeMode=uint8
  Direction Cosine Matrix to Euler Angles : Subsystem  AncestorBlock=aerolibtransform2/Direction Cosine Matrix to Euler Angles  mask(DCM2Euler){}
      mask help: Determine an euler orientation (roll, pitch, yaw) from the 3-by-3 direction cosine matrix (DCM). The input DCM transforms vectors from geodetic earth or north-down-east (NED) axes to body axes.
      mask init:
      | aeroicon('aeroblk');
      mask Help: web(asbhelp('directioncosinematrixtoeulerangles'));
      mask Display:
      | port_label('output',1,'\phi','texmode','on')
      | port_label('output',2,'\theta','texmode','on')
      | port_label('output',3,'\psi','texmode','on')
      | port_label('input',1,'DCM_{be}','texmode','on')
  Embedded MATLAB Function : Stateflow chart
  Euler : Selector  IndexOptions=Index vector (dialog)  Indices=[1 2 3]  OutputSizes=1  InputPortWidth=6
  Euler Angles to  Direction Cosine Matrix1 : Subsystem  AncestorBlock="aerolibtransform2/Euler Angles to  Direction Cosine Matrix"  mask(Euler2DCM){}
      mask help: Determine the 3-by-3 direction cosine matrix (DCM) from an Euler orientation (roll, pitch, yaw). The output DCM transforms vectors from geodetic earth or north-east-down (NED) axes to body axes.
      mask init:
      | aeroicon('aeroblk');
      mask Help: web(asbhelp('euleranglestodirectioncosinematrix'));
      mask Display:
      | port_label('input',1,'\phi \theta \psi','texmode','on')
      | port_label('output',1,'DCM_{be}','texmode','on')
  Euler Angles to  Direction Cosine Matrix2 : Subsystem  AncestorBlock="aerolibtransform2/Euler Angles to  Direction Cosine Matrix"  mask(Euler2DCM){}
      mask help: Determine the 3-by-3 direction cosine matrix (DCM) from an Euler orientation (roll, pitch, yaw). The output DCM transforms vectors from geodetic earth or north-east-down (NED) axes to body axes.
      mask init:
      | aeroicon('aeroblk');
      mask Help: web(asbhelp('euleranglestodirectioncosinematrix'));
      mask Display:
      | port_label('input',1,'\phi \theta \psi','texmode','on')
      | port_label('output',1,'DCM_{be}','texmode','on')
  Get Attitude [navSupport.c] : dsPICdrivers/OTHERS/C Function Call  Tag=dsPIC_dsPIC_CFunctionCall  fctName='getAttitude'  INPUT_SIZE=1  INPUT1=--  INPUT2=--  INPUT3=--  OUTPUT_SIZE=6  OUTPUT1=real32  SampleTime=.01  InputType=[ ]  OutputType=[ 7 ]  FctDeclaration=extern void getAttitude(real32_T* y1);  FctCall=getAttitude(*%y1);  OrderingInOutPopup=None
  Get the Accel Bias [navSupport.c] : dsPICdrivers/OTHERS/C Function Call  Tag=dsPIC_dsPIC_CFunctionCall  fctName='getAccBias'  INPUT_SIZE=1  INPUT1=--  INPUT2=--  INPUT3=--  OUTPUT_SIZE=3  OUTPUT1=real32  SampleTime=.01  InputType=[ ]  OutputType=[ 7 ]  FctDeclaration=extern void getAccBias(real32_T* y1);  FctCall=getAccBias(*%y1);  OrderingInOutPopup=None
  Get the Accelerometers [navSupport.c] : dsPICdrivers/OTHERS/C Function Call  Tag=dsPIC_dsPIC_CFunctionCall  fctName='getAccels'  INPUT_SIZE=1  INPUT1=--  INPUT2=--  INPUT3=--  OUTPUT_SIZE=3  OUTPUT1=real32  SampleTime=.01  InputType=[ ]  OutputType=[ 7 ]  FctDeclaration=extern void getAccels(real32_T* y1);  FctCall=getAccels(*%y1);  OrderingInOutPopup=None
  Math Function : Math  Operator=transpose  SaturateOnIntegerOverflow=on
  Product{,1..3} (4 alike) : Product  Multiplication=Matrix(*)  RndMeth=Zero
  Rates : Selector  IndexOptions=Index vector (dialog)  Indices=[4 5 6]  OutputSizes=1  InputPortWidth=6
  Selector : Selector  IndexOptions=Index vector (dialog)  Indices=[1 2 5 6]  OutputSizes=1  InputPortWidth=6
  Selector1 : Selector  IndexOptions=Index vector (dialog)  Indices=[2]  OutputSizes=1  InputPortWidth=3
  Sum : Sum  Inputs=+|+
  "[navSupport.c] " : dsPICdrivers/OTHERS/C Function Call  Tag=dsPIC_dsPIC_CFunctionCall  fctName='getPidIdx'  INPUT_SIZE=1  INPUT1=uint8  INPUT2=--  INPUT3=--  OUTPUT_SIZE=3  OUTPUT1=real32  SampleTime=.01  InputType=[ 2 ]  OutputType=[ 7 ]  FctDeclaration=extern void getPidIdx(uint8_T u1,real32_T* y1);  FctCall=getPidIdx(%u1, *%y1);  OrderingInOutPopup=None
  myMux Fun1 : Stateflow chart
  myMux Fun2 : Stateflow chart
  "[phi the q r]" : Outport
  Euler Rot : Outport  Port=2
  PQR Rot : Outport  Port=3
  Yb Accel : Outport  Port=4
  wires:
  Constant2/1 -> "[navSupport.c] "/1
  Selector/1 -> "[phi the q r]"/1
  Get Attitude [navSupport.c]/1 -> Euler/1, Rates/1
  Euler/1 -> Euler Angles to  Direction Cosine Matrix2/1(Euler Roll Pitch Yaw)
  Euler Angles to  Direction Cosine Matrix2/1(DCM) -> Product/2
  "[navSupport.c] "/1 -> Angle Conversion/1
  Euler Angles to  Direction Cosine Matrix1/1(DCM) -> Math Function/1
  Angle Conversion/1 -> Euler Angles to  Direction Cosine Matrix1/1(Euler Roll Pitch Yaw)
  Direction Cosine Matrix to Euler Angles/3(psi) -> Embedded MATLAB Function/1(u)
  Direction Cosine Matrix to Euler Angles/1(phi) -> myMux Fun1/1(u1)
  Direction Cosine Matrix to Euler Angles/2(theta) -> myMux Fun1/2(u2)
  Embedded MATLAB Function/1(y) -> myMux Fun1/3(u3)
  Product/1 -> Direction Cosine Matrix to Euler Angles/1(DCM)
  Rates/1 -> Product1/2
  myMux Fun1/1(y) -> Euler Rot/1, myMux Fun2/1(u1)
  Product1/1 -> myMux Fun2/2(u2), PQR Rot/1
  myMux Fun2/1(y) -> Selector/1
  Math Function/1 -> Product/1, Product1/1, Product2/1, Product3/1
  Get the Accelerometers [navSupport.c]/1 -> Product2/2
  Get the Accel Bias [navSupport.c]/1 -> Product3/2
  Product2/1 -> Sum/1
  Product3/1 -> Sum/2
  Sum/1 -> Selector1/1
  Selector1/1 -> Yb Accel/1

== system controlMCUSlugsMKII/Data  Sources/Compute Load ==
  Calculus Time Step : dsPICdrivers/OTHERS/Calculus Time Step  Tag=dsPIC_CalculusTimeStep  SampleTime=0.01  PR1chk=on
  Data Type Conversion12 : DataTypeConversion  OutDataTypeMode=uint8
  Data Type Conversion3 : DataTypeConversion  OutDataTypeMode=single
  Data Type Conversion4 : DataTypeConversion  OutDataTypeMode=single
  Divide : Product  Inputs=*/  OutDataTypeMode=double  OutScaling=2^-10
  Gain : Gain  Gain=100
  Rounding Function : Rounding
  Load (%) : Outport
  wires:
  Calculus Time Step/1 -> Data Type Conversion4/1
  Calculus Time Step/2 -> Data Type Conversion3/1
  Divide/1 -> Gain/1
  Rounding Function/1 -> Data Type Conversion12/1
  Data Type Conversion3/1 -> Divide/2
  Data Type Conversion4/1 -> Divide/1
  Data Type Conversion12/1 -> Load (%)/1
  Gain/1 -> Rounding Function/1

== system controlMCUSlugsMKII/Inner Loop/ Navigation/Compute psi_dot_m ==
  r_m : Inport
  phi_m : Inport  Port=2
  q_m : Inport  Port=3
  Product : Product  SampleTime=apSampleTime  RndMeth=Zero
  Product1 : Product  SampleTime=apSampleTime  RndMeth=Zero
  Protect NaNs : Subsystem
  Subsystem5 : Subsystem  AncestorBlock=SLUGS_Library/Subsystem5
  Subsystem7 : Subsystem  AncestorBlock=SLUGS_Library/Subsystem7
  Subtract : Sum  Inputs=2  OutScaling=2^-10
  psi_dot_m : Outport
  wires:
  q_m/1 -> Product1/1
  Subtract/1 -> Protect NaNs/1(In1)
  phi_m/1 -> Subsystem7/1(x), Subsystem5/1(u)
  r_m/1 -> Product/1
  Product1/1 -> Subtract/2
  Product/1 -> Subtract/1
  Subsystem7/1(sin(x)) -> Product1/2
  Subsystem5/1(cos(u)) -> Product/2
  Protect NaNs/1(Out1) -> psi_dot_m/1

== system controlMCUSlugsMKII/Inner Loop/ Navigation/L1 Output Feedback Controller With  Projection Operator ==
  psi_dot_m : Inport
  m : Inport  Port=2
  omega : Inport  Port=3
  gamma : Inport  Port=4
  psi_dot_c : Inport  Port=5
  Enable : EnablePort  StatesWhenEnabling=reset  ShowOutputPort=on
  Constant : Constant  Value=2  OutDataTypeMode=single
  Constant1 : Constant  OutDataTypeMode=single
  Control  Law : Subsystem
      mask Display:
      | droots([],'-a','a')
      | port_label('input',1,'a')
      | port_label('input',2,'u')
      | port_label('output',1,'y')
  Gain : Gain  Gain=-1
  Integer Delay : simulink/Discrete/Integer Delay  vinit=0.0  samptime=.01  NumDelays=1
  Integer Delay1 : simulink/Discrete/Integer Delay  Orientation=left  vinit=0.0  samptime=.01  NumDelays=1
  Logical Operator : Logic  Operator=NOT  AllPortsSameDT=off  OutDataTypeMode=Specify via dialog
  Projection : Product  OutDataTypeMode=single  SampleTime=apSampleTime  RndMeth=Zero
  Projection Operator : Subsystem
  Protect NaNs : Subsystem
  Protect NaNs2 : Subsystem
  Psi Dot  Limit : Saturate  UpperLimit=1  LowerLimit=-1  SampleTime=apSampleTime
  State Predictor : Subsystem
      mask Display:
      | droots([],'-a','a')
      | port_label('input',1,'a')
      | port_label('input',2,'u')
      | port_label('output',1,'y')
  Sum2 : Sum  Inputs=|++  OutDataTypeMode=single  SampleTime=apSampleTime
  Sum3 : Sum  Inputs=-+|  OutDataTypeMode=single  SampleTime=apSampleTime
  Sum4 : Sum  Inputs=+-|  OutDataTypeMode=single  SampleTime=apSampleTime
  Trapezoidal Integrator : Subsystem  AncestorBlock=SLUGS_Library/Control Blocks/PID Controller w//Anti-Windup/Trapezoidal Integrator  mask{T=apSampleTime, upperLimit=2, lowerLimit=-2}
      mask prompts: T "Sample Time"; upperLimit "Upper Saturation"; lowerLimit "Lower Saturation"
  psi_dot_ad : Outport
  wires:
  Integer Delay/1 -> Sum4/1  "psi_dot_c"
  State Predictor/1(y) -> Sum3/2
  Gain/1 -> Projection Operator/4(y)
  m/1 -> State Predictor/1(a)
  Sum2/1 -> Protect NaNs2/1(In1)
  psi_dot_m/1 -> Protect NaNs/1(In1)  "psi_dot_m"
  Sum3/1 -> Gain/1  "psi_dot_tilde"
  gamma/1 -> Projection/1  "adaptation gain"
  Projection/1 -> Trapezoidal Integrator/1(x)
  psi_dot_c/1 -> Integer Delay/1  "psi_dot_c"
  omega/1 -> Control  Law/1(a)
  Control  Law/1(y) -> Sum4/2  "sigma_hat_fil"
  Sum4/1 -> Psi Dot  Limit/1  "psi_ad"
  Projection Operator/1("Proj(the, y)") -> Projection/2  "Proj"
  Constant/1 -> Projection Operator/1(Theta Max)
  Constant1/1 -> Projection Operator/2(Eps 0)
  Integer Delay1/1 -> Sum2/2, Projection Operator/3(Theta)
  Enable/1 -> Logical Operator/1
  Logical Operator/1 -> Trapezoidal Integrator/2(Reset)
  Trapezoidal Integrator/1(Int(x)) -> Control  Law/2(u), Integer Delay1/1  "sigma_hat"
  Protect NaNs2/1(Out1) -> State Predictor/2(u)
  Protect NaNs/1(Out1) -> Sum3/1
  Psi Dot  Limit/1 -> psi_dot_ad/1, Sum2/1

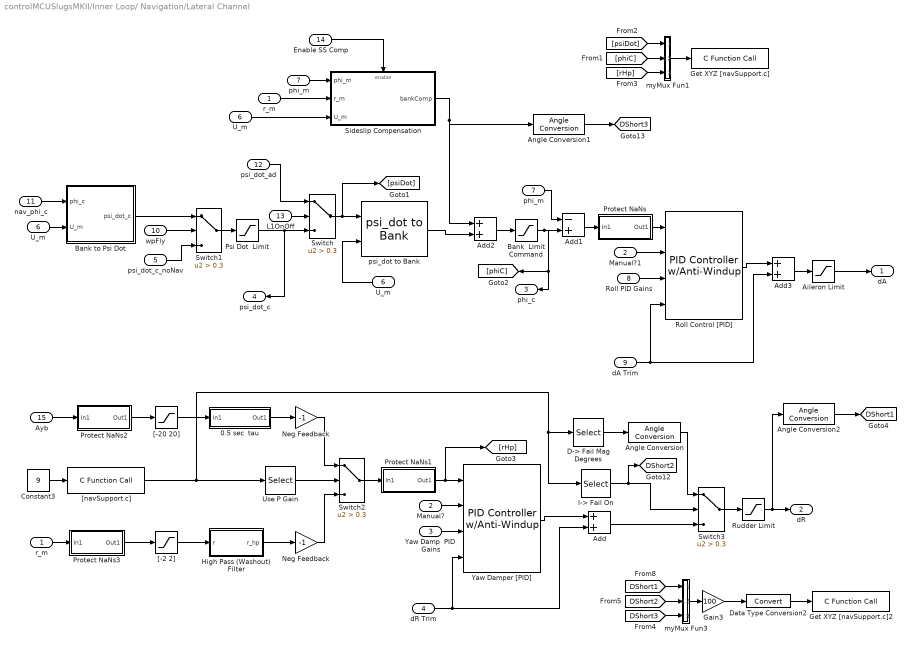
== system controlMCUSlugsMKII/Inner Loop/ Navigation/Lateral Channel ==
  r_m : Inport
  Manual? : Inport  Port=2
  Yaw Damp  PID Gains : Inport  Port=3
  dR Trim : Inport  Port=4
  psi_dot_c_noNav : Inport  Port=5
  U_m : Inport  Port=6
  phi_m : Inport  Port=7
  Roll PID Gains : Inport  Port=8
  dA Trim : Inport  Port=9
  wpFly : Inport  Port=10  SampleTime=apSampleTime
  nav_phi_c : Inport  Port=11
  psi_dot_ad : Inport  Port=12  SampleTime=apSampleTime
  L1OnOff : Inport  Port=13
  Enable SS Comp : Inport  Port=14
  Ayb : Inport  Port=15
  0.5 sec  tau : Subsystem  mask(Tustin1stOrderLowpassAutoInitialCondition){f=0.3183, T=T}
      mask prompts: f "Lowpass Frequency"; T "Sample Time"
      mask help: Takes a 3db rolloff frequency (in Hz, NOT radians/s) and a sample time. Performs a symbolic Tustin conversion and implements in a discrete filter. The initial output of the filter is set by the first sample.
      mask Help: Enter the desired 3db rolloff frequency in Hz and the sample time. Initial conditions are sampled automatically.
      mask Display: fprintf('%.2f Hz lowpass',f)
  Add : Sum  OutDataTypeMode=single  OutScaling=2^-10
  Add1 : Sum  Inputs=-+  OutDataTypeMode=single  OutScaling=2^-10
  Add2 : Sum  OutDataTypeMode=single  OutScaling=2^-10
  Add3 : Sum  OutDataTypeMode=single  OutScaling=2^-10
  Aileron Limit : Saturate  UpperLimit=daLimit  LowerLimit=-daLimit  SampleTime=apSampleTime
  Angle Conversion : aerolibconvert2/Angle Conversion  SystemSampleTime=-1  IU=deg  OU=rad
  Angle Conversion1 : aerolibconvert2/Angle Conversion  SystemSampleTime=-1  IU=rad  OU=deg
  Angle Conversion2 : aerolibconvert2/Angle Conversion  SystemSampleTime=-1  IU=rad  OU=deg
  Bank  Limit Command : Saturate  UpperLimit=bankCommandLimit  LowerLimit=-bankCommandLimit  SampleTime=apSampleTime
  Bank to Psi Dot : Subsystem  AncestorBlock=SLUGS_Library/Navigation/Bank to Psi Dot
  Constant3 : Constant  Value=9  OutDataTypeMode=uint8
  D-> Fail Mag Degrees : Selector  IndexOptions=Index vector (dialog)  Indices=3  OutputSizes=1  InputPortWidth=3
  Data Type Conversion2 : DataTypeConversion  OutDataTypeMode=int16
  Gain3 : Gain  Gain=100  OutDataTypeMode=Specify via dialog  OutDataType=float('single')
  Get XYZ [navSupport.c] : dsPICdrivers/OTHERS/C Function Call  Tag=dsPIC_dsPIC_CFunctionCall  fctName='setNavLat'  INPUT_SIZE=3  INPUT1=real32  INPUT2=--  INPUT3=--  OUTPUT_SIZE=1  OUTPUT1=--  SampleTime=.01  InputType=[ 7 ]  OutputType=[ ]  FctDeclaration=extern void setNavLat(real32_T* u1);  FctCall=setNavLat(*%u1);  OrderingInOutPopup=None
  Get XYZ [navSupport.c]2 : dsPICdrivers/OTHERS/C Function Call  Tag=dsPIC_dsPIC_CFunctionCall  fctName='setDiagnosticShort'  INPUT_SIZE=3  INPUT1=int16  INPUT2=--  INPUT3=--  OUTPUT_SIZE=1  OUTPUT1=--  SampleTime=.01  InputType=[ 3 ]  OutputType=[ ]  FctDeclaration=extern void setDiagnosticShort(int16_T* u1);  FctCall=setDiagnosticShort(*%u1);  OrderingInOutPopup=None
  High Pass (Washout) Filter : Subsystem  TreatAsAtomicUnit=on
  I-> Fail On : Selector  IndexOptions=Index vector (dialog)  Indices=2  OutputSizes=1  InputPortWidth=3
  Manual?1 : InportShadow  Port=2  LatchByCopyingInsideSignal=off
  Neg Feedback : Gain  Gain=-1  OutDataTypeMode=Specify via dialog  OutDataType=float('single')
  "Neg Feedback " : Gain  Gain=-1  OutDataTypeMode=Specify via dialog  OutDataType=float('single')
  Protect NaNs : Subsystem
  Protect NaNs1 : Subsystem
  Protect NaNs2 : Subsystem
  Protect NaNs3 : Subsystem
  Psi Dot  Limit : Saturate  UpperLimit=1  LowerLimit=-1  SampleTime=apSampleTime
  Roll Control [PID] : SLUGS_Library/Control Blocks/PID Controller w//Anti-Windup  SystemSampleTime=-1  Tsample=apSampleTime  Ndelay=derivativesConstant  upperSaturationLimit=daLimit  lowerSaturationLimit=-daLimit
  Rudder Limit : Saturate  UpperLimit=drLimit  LowerLimit=-drLimit  SampleTime=apSampleTime
  Sideslip Compensation : Subsystem
  Switch : Switch  Criteria=u2 > Threshold  Threshold=0.3
  Switch1 : Switch  Criteria=u2 > Threshold  Threshold=0.3  InputSameDT=on
  Switch2 : Switch  Criteria=u2 > Threshold  Threshold=0.3
  Switch3 : Switch  Criteria=u2 > Threshold  Threshold=0.3
  "U_m  " : InportShadow  Orientation=left  Port=6  LatchByCopyingInsideSignal=off
  "U_m   " : InportShadow  Port=6  LatchByCopyingInsideSignal=off
  Use P Gain : Selector  IndexOptions=Index vector (dialog)  Indices=1  OutputSizes=1  InputPortWidth=3
  Yaw Damper [PID] : SLUGS_Library/Control Blocks/PID Controller w//Anti-Windup  SystemSampleTime=-1  Tsample=apSampleTime  Ndelay=derivativesConstant  upperSaturationLimit=drLimit  lowerSaturationLimit=-drLimit
  "[-2 2]" : Saturate  UpperLimit=2  LowerLimit=-2
  "[-20 20]" : Saturate  UpperLimit=20  LowerLimit=-20
  "[navSupport.c]   " : dsPICdrivers/OTHERS/C Function Call  Tag=dsPIC_dsPIC_CFunctionCall  fctName='getPidIdx'  INPUT_SIZE=1  INPUT1=uint8  INPUT2=--  INPUT3=--  OUTPUT_SIZE=3  OUTPUT1=real32  SampleTime=.01  InputType=[ 2 ]  OutputType=[ 7 ]  FctDeclaration=extern void getPidIdx(uint8_T u1,real32_T* y1);  FctCall=getPidIdx(%u1, *%y1);  OrderingInOutPopup=None
  myMux Fun1 : Stateflow chart
  myMux Fun3 : Stateflow chart
  "phi_m  " : InportShadow  Port=7  LatchByCopyingInsideSignal=off
  psi_dot to Bank : SLUGS_Library/Navigation/psi_dot to Bank  SystemSampleTime=-1
  "r_m  " : InportShadow  Port=1  LatchByCopyingInsideSignal=off
  dA : Outport
  dR : Outport  Port=2
  phi_c : Outport  Orientation=left  Port=3
  "psi_dot_c " : Outport  Orientation=left  Port=4
  tag scope: DShort1=global, DShort2=global, DShort3=global
  wires:
  nav_phi_c/1 -> Bank to Psi Dot/1(phi_c)
  Bank  Limit Command/1 -> Add1/2, [phiC], phi_c/1
  phi_m/1 -> Add1/1
  Add1/1 -> Protect NaNs/1(In1)
  Aileron Limit/1 -> dA/1
  dA Trim/1 -> Add3/2, Roll Control [PID]/4
  Roll Control [PID]/1 -> Add3/1
  Add3/1 -> Aileron Limit/1
  Roll PID Gains/1 -> Roll Control [PID]/3
  Manual?1/1 -> Roll Control [PID]/2
  U_m/1 -> Bank to Psi Dot/2(U_m)
  dR Trim/1 -> Add/2, Yaw Damper [PID]/4
  Yaw Damper [PID]/1 -> Add/1
  Add/1 -> Switch3/3
  Yaw Damp  PID Gains/1 -> Yaw Damper [PID]/3
  Manual?/1 -> Yaw Damper [PID]/2
  r_m/1 -> Protect NaNs3/1(In1)
  Switch/1 -> psi_dot to Bank/1, [psiDot]
  Switch1/1 -> Psi Dot  Limit/1
  L1OnOff/1 -> Switch/2
  psi_dot_ad/1 -> Switch/1
  wpFly/1 -> Switch1/2
  psi_dot_c_noNav/1 -> Switch1/3
  Bank to Psi Dot/1(psi_dot_c) -> Switch1/1
  "U_m  "/1 -> psi_dot to Bank/2
  "[-2 2]"/1 -> High Pass (Washout) Filter/1(r)
  myMux Fun1/1(y) -> Get XYZ [navSupport.c]/1
  [psiDot] -> myMux Fun1/1(u1)
  [phiC] -> myMux Fun1/2(u2)
  [rHp] -> myMux Fun1/3(u3)
  Add2/1 -> Bank  Limit Command/1
  psi_dot to Bank/1 -> Add2/2
  Sideslip Compensation/1(bankComp) -> Add2/1, Angle Conversion1/1
  "phi_m  "/1 -> Sideslip Compensation/1(phi_m)
  "r_m  "/1 -> Sideslip Compensation/2(r_m)
  "U_m   "/1 -> Sideslip Compensation/3(U_m)
  Enable SS Comp/1 -> Sideslip Compensation/Enable
  Switch2/1 -> Protect NaNs1/1(In1)
  High Pass (Washout) Filter/1(r_hp) -> Neg Feedback/1
  Ayb/1 -> Protect NaNs2/1(In1)
  Constant3/1 -> "[navSupport.c]   "/1
  "[navSupport.c]   "/1 -> Use P Gain/1, I-> Fail On/1, D-> Fail Mag Degrees/1
  Use P Gain/1 -> Switch2/2
  "Neg Feedback "/1 -> Switch2/1
  0.5 sec  tau/1(Out1) -> "Neg Feedback "/1
  Switch3/1 -> Rudder Limit/1
  I-> Fail On/1 -> Switch3/2, [DShort2]
  D-> Fail Mag Degrees/1 -> Angle Conversion/1
  Angle Conversion/1 -> Switch3/1
  Rudder Limit/1 -> dR/1, Angle Conversion2/1
  [DShort1] -> myMux Fun3/1(u1)
  [DShort2] -> myMux Fun3/2(u2)
  [DShort3] -> myMux Fun3/3(u3)
  myMux Fun3/1(y) -> Gain3/1
  Gain3/1 -> Data Type Conversion2/1
  Data Type Conversion2/1 -> Get XYZ [navSupport.c]2/1
  Angle Conversion1/1 -> [DShort3]
  Angle Conversion2/1 -> [DShort1]
  Protect NaNs/1(Out1) -> Roll Control [PID]/1
  Protect NaNs1/1(Out1) -> [rHp], Yaw Damper [PID]/1
  Protect NaNs2/1(Out1) -> "[-20 20]"/1
  Protect NaNs3/1(Out1) -> "[-2 2]"/1
  "[-20 20]"/1 -> 0.5 sec  tau/1(In1)
  Neg Feedback/1 -> Switch2/3
  Psi Dot  Limit/1 -> Switch/3, "psi_dot_c "/1
